simulink model "lame2"  (R2019b)
settings: Solver=VariableStepAuto  StartTime=0.0  StopTime=1  RelTol=1e-3
model workspace (MAT data in the model file):
  E = 16950000000
  J = 2.4620533875e-11
  L = 0.27
  dens = 1909.91
  dt = 7e-05
  dx = 0.0675
  g = 9.81
  gamma = 0.15
  h = 0.00159
  l = 0.0735
  mu = 0.22320163215
  nx = 20
  w = [0 0 0 0 0 0 0 0 0 0 0 0 0 0 0 0 0 0 0 0]
settings Model: OrderedModelArguments=off  Creator=MAGUY18  LastModifiedBy=frfoc1
settings SolverCC: AlgebraicLoopSolver=LineSearch

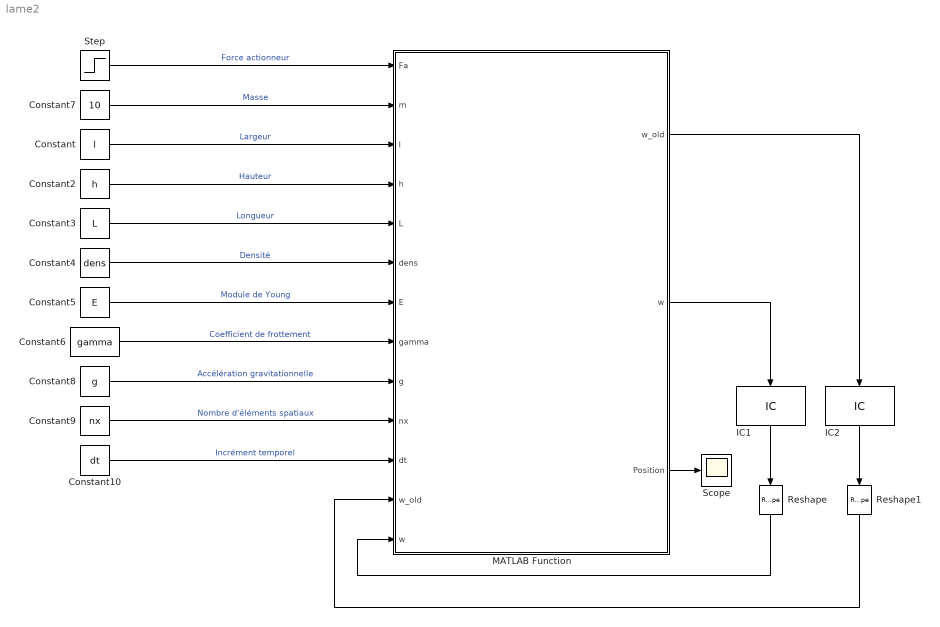
== system lame2 ==
  Constant : Constant  Value=l
  Constant10 : Constant  Value=dt
  Constant2 : Constant  Value=h
  Constant3 : Constant  Value=L
  Constant4 : Constant  Value=dens
  Constant5 : Constant  Value=E
  Constant6 : Constant  Value=gamma
  Constant7 : Constant  Value=10
  Constant8 : Constant  Value=g
  Constant9 : Constant  Value=nx
  IC1 : InitialCondition  Value=zeros(1, nx)
  IC2 : InitialCondition  Value=zeros(1, nx)
  MATLAB Function : MATLAB Function  TreatAsAtomicUnit=on  SystemSampleTime=dt
  Reshape : Reshape  OutputDimensionality=Row vector (2-D)
  Reshape1 : Reshape  OutputDimensionality=Row vector (2-D)
  Scope : Scope
  Step : Step  Time=0  After=0.5  SampleTime=dt
  wires:
  Step/1 -> MATLAB Function/1(Fa)  "Force actionneur"
  Constant/1 -> MATLAB Function/3(l)  "Largeur"
  Constant2/1 -> MATLAB Function/4(h)  "Hauteur"
  Constant3/1 -> MATLAB Function/5(L)  "Longueur"
  Constant4/1 -> MATLAB Function/6(dens)  "Densité"
  Constant5/1 -> MATLAB Function/7(E)  "Module de Young"
  Constant6/1 -> MATLAB Function/8(gamma)  "Coefficient de frottement"
  Constant7/1 -> MATLAB Function/2(m)  "Masse"
  Constant8/1 -> MATLAB Function/9(g)  "Accélération gravitationnelle"
  Constant9/1 -> MATLAB Function/10(nx)  "Nombre d'éléments spatiaux"
  Constant10/1 -> MATLAB Function/11(dt)  "Incrément temporel"
  MATLAB Function/3(Position) -> Scope/1
  MATLAB Function/1(w_old) -> IC2/1
  MATLAB Function/2(w) -> IC1/1
  IC1/1 -> Reshape/1
  IC2/1 -> Reshape1/1
  Reshape/1 -> MATLAB Function/13("w ")
  Reshape1/1 -> MATLAB Function/12("w_old ")

== matlab function lame2/MATLAB Function ==
  data: w_old output; Fa input; m input; l input; h input; L input; dens input; E input; gamma input; g input; nx input; dt input; w_old input; w input; w output; Position output
function [w_old, w, Position]= fcn(Fa, m, l, h, L, dens, E, gamma, g, nx, dt, w_old, w)

J = l*h^3/12;      
mu =  dens*l*h;
poids = (m/1000) * g;

dx = L/(nx-1);
x  = (0:dx:L);

force_actionneur = [0 0 0 0 0 0 0 0 0 0 0 0 0 0 0 0 0 0 0 0]; %Array sous cette forme car la fonction zeros(1, nx) marche pas
force_actionneur(13) = Fa;

force_grav = [0 0 0 0 0 0 0 0 0 0 0 0 0 0 0 0 0 0 0 0];
force_grav(13) = poids;

%Loop

w_new = [0 0 0 0 0 0 0 0 0 0 0 0 0 0 0 0 0 0 0 0];

i = 3:nx-2; % à partir de 3 comme ça 1 et 2 reste à 0 toujours

w_new(i) = (1/((mu/dt^2)+(gamma/(2*dt)))) * ((mu/dt^2)*(2*w(i)-w_old(i)) + gamma*w_old(i)/(2*dt) - ...
    (E*J/dx^4)*(w(i+2) - 4*w(i+1) + 6*w(i) - 4*w(i-1) + w(i-2)) + (force_actionneur(i)-force_grav(i))/dx);

w_new(1:2) = 0; % Clampé à zero, position et dérivée nulle des deux premiers éléments


w_new(end-1) = 2*w_new(end-2)-w_new(end-3);    % Libre au bout dérivées 2e et 3e nulles
w_new(end) = 2*w_new(end-1)-w_new(end-2);

w_old=w;
w = w_new;

Position = w(18);
